simulink model "gnc_dst"  (R2023a)
settings: Solver=ode4  StartTime=0.0  StopTime=10.0  FixedStep=dt  RelTol=1e-3
undefined symbols (not defined in the file or in its folder): dt, plant, roe_mat, u_mat_full, u_time
libraries: aerolibutil x2
settings Model: Creator=ndelurgio  LastModifiedBy=ndelurgio
settings DebuggingCC: ModelReferenceExtraNoncontSigs=none

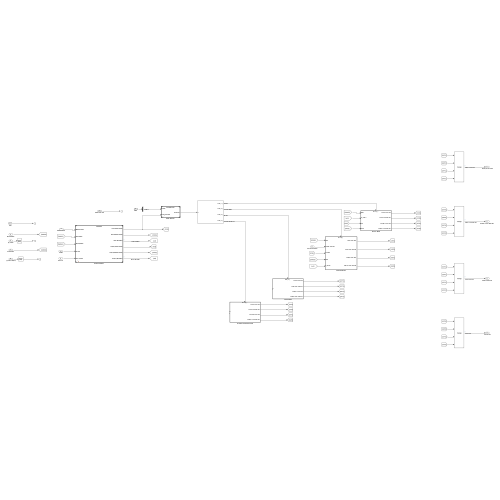
[thumbnail: Simulink's stored preview of the top-level diagram]
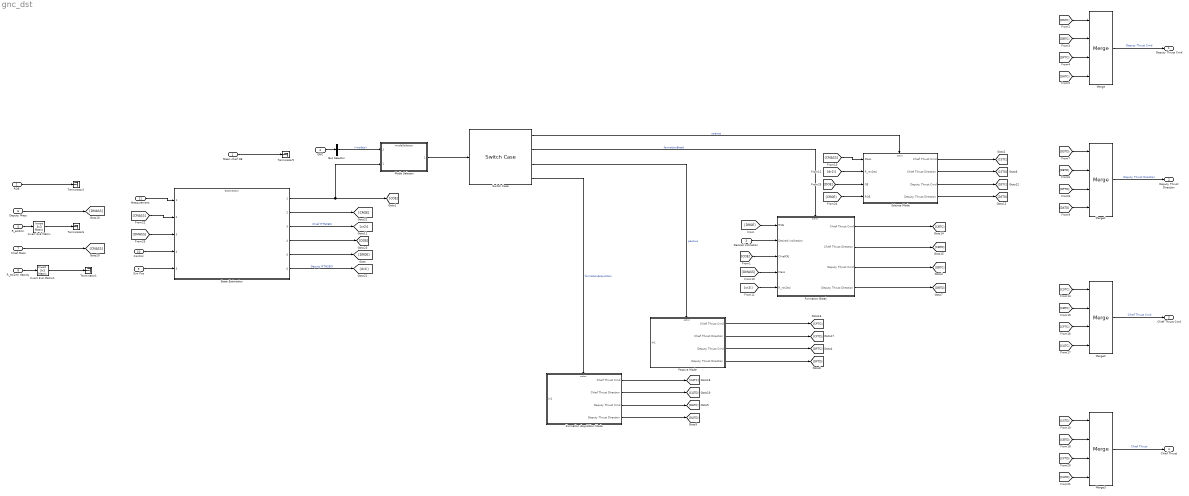
== system gnc_dst ==
  Mean chief OE : Inport  OutDataTypeStr=Bus: meanOrbitElements
  ROE : Inport  Port=2  OutDataTypeStr=Bus: eccentricSingularROE
  Desired inclination : Inport  Port=3  PortDimensions=2
  GNC : Inport  Port=4  OutDataTypeStr=Bus: gncBus
  R_eci2rtn : Inport  Port=5  PortDimensions=[3,3]
  Deputy Mass : Inport  Port=6
  Chief Mass : Inport  Port=7
  R_eci2rtn deputy : Inport  Port=8
  Sun Pos : Inport  Port=9
  Control : Inport  Port=10
  Measurement : Inport  Port=11
  Bus Selector : BusSelector  OutputSignals=modes
  Formation Acquisition Mode : Subsystem  TreatAsAtomicUnit=on
  Formation Break : Subsystem  TreatAsAtomicUnit=on
  Invert 3x3 Matrix : aerolibutil/Invert  3x3 Matrix
  Invert 3x3 Matrix1 : aerolibutil/Invert  3x3 Matrix
  Merge : Merge  Inputs=4  InitialOutput=0
  Merge1 : Merge  Inputs=4  InitialOutput=[1,1,1]
  Merge2 : Merge  Inputs=4  InitialOutput=0
  Merge3 : Merge  Inputs=4  InitialOutput=[1,1,1]
  Mode Selector : ModelReference  ModelNameDialog=modeSelector.slx  SimulationMode=Normal  ModelReferenceVersion=1.18
      settings: PortSchema="{\"entries\":[{\"content\":{\"sides\":[{\"content\":{\"connectorIds\":[\"In2\",\"In1\"]},\"type\":\"ConnectorPlacement.EquallySpacedRectSide\",\"uuid\":\"8a45dd05-9625-4267-a143-38565687985f\"},{\"content\":{\"connectorIds\":[\"Out1\"],\"side\":\"RIGHT\"},\"type\":\"ConnectorPlacement.EquallySpacedRectSide\",\"uuid\":\"c16609dd-c717-4d96-a97d-40d34aa61c5b\"},{\"content\":{\"side\":\"TOP\"},\"type\":\"ConnectorPlacement.EquallySpacedRectSide\",\"uuid\":\"265a618d-b5cc-4228-aeff-cbf882e13e2d\"}]},\"type\":\"ConnectorPlacement.EquallySpacedConnector\",\"uuid\":\"354b4fb0-049b-4d87-9ce4-a2a1b71aacc7\"}],\"packageUris\":[\"http://schema.mathworks.com/mf0/Connector/R2020b\"],\"version\":\"1.0\"}"
  Passive Mode : Subsystem  TreatAsAtomicUnit=on
  Science Mode : Subsystem  TreatAsAtomicUnit=on
  State Estimation : ModelReference  ModelNameDialog=estimation.slx  SimulationMode=Normal  ModelReferenceVersion=1.37
  Switch Case : SwitchCase  CaseConditions={1,2,3,4}  ShowDefaultCase=off
  Terminator{1..2,5..6} (4 alike) : Terminator
  Deputy Thrust Cmd : Outport
  Deputy Thrust Direction : Outport  Port=2
  Chief Thrust Cmd : Outport  Port=3
  Chief Thrust : Outport  Port=4
  wires:
  Mean chief OE/1 -> Terminator5/1
  ROE/1 -> Terminator2/1
  Desired inclination/1 -> Formation Break/2(Desired inclination)
  Merge/1 -> Deputy Thrust Cmd/1  "Deputy Thrust Cmd"
  Merge1/1 -> Deputy Thrust Direction/1  "Deputy Thrust Direction"
  Switch Case/1 -> Science Mode/Action  "science"
  Switch Case/2 -> Formation Break/Action  "formationBreak"
  Switch Case/3 -> Passive Mode/Action  "passive"
  Switch Case/4 -> Formation Acquisition Mode/Action  "formationAcquisition"
  Mode Selector/1 -> Switch Case/1
  GNC/1 -> Bus Selector/1
  Bus Selector/1 -> Mode Selector/2  "<modes>"
  [DROE] -> Formation Break/1(ROE)
  [COE] -> Formation Break/3(ChiefOE)
  Invert 3x3 Matrix/1 -> Terminator6/1
  Deputy Mass/1 -> [DMASS]
  R_eci2rtn/1 -> Invert 3x3 Matrix/1
  Science Mode/1(Chief Thrust Cmd) -> [CSTC]
  Formation Break/3(Deputy Thrust Cmd) -> [DBTC]
  Passive Mode/3(Deputy Thrust Cmd) -> [DPTC]
  Formation Acquisition Mode/3(Deputy Thrust Cmd) -> [DATC]
  [DSTC] -> Merge/1
  [DBTC] -> Merge/2
  [DPTC] -> Merge/3
  [DATC] -> Merge/4
  Science Mode/2(Chief Thrust Direction) -> [CSTD]
  Formation Break/4(Deputy Thrust Direction) -> [DBTD]
  Passive Mode/4(Deputy Thrust Direction) -> [DPTD]
  Formation Acquisition Mode/4(Deputy Thrust Direction) -> [DATD]
  [DSTD] -> Merge1/1
  [DBTD] -> Merge1/2
  [DPTD] -> Merge1/3
  [DATD] -> Merge1/4
  [DMASS] -> Formation Break/4(Mass)
  [cr2i] -> Formation Break/5(R_rtn2eci)
  [dr2i] -> Science Mode/2(R_rtn2eci)
  [CMASS] -> Science Mode/1(Mass)
  Science Mode/3(Deputy Thrust Cmd) -> [DSTC]
  Science Mode/4(Deputy Thrust Direction) -> [DSTD]
  Formation Break/2(Chief Thrust Direction) -> [CBTD]
  Formation Break/1(Chief Thrust Cmd) -> [CBTC]
  Passive Mode/1(Chief Thrust Cmd) -> [CPTC]
  Passive Mode/2(Chief Thrust Direction) -> [CPTD]
  Formation Acquisition Mode/1(Chief Thrust Cmd) -> [CATC]
  Formation Acquisition Mode/2(Chief Thrust Direction) -> [CATD]
  [CSTC] -> Merge2/1
  [CPTC] -> Merge2/3
  [CATC] -> Merge2/4
  [CBTC] -> Merge2/2
  [CSTD] -> Merge3/1
  [CBTD] -> Merge3/2
  [CATD] -> Merge3/4
  [CPTD] -> Merge3/3
  Merge3/1 -> Chief Thrust/1  "Chief Thrust"
  Merge2/1 -> Chief Thrust Cmd/1  "Chief Thrust Cmd"
  Chief Mass/1 -> [CMASS]
  R_eci2rtn deputy/1 -> Invert 3x3 Matrix1/1
  Invert 3x3 Matrix1/1 -> Terminator1/1
  [CMASS] -> State Estimation/2
  [DMASS] -> State Estimation/3
  Sun Pos/1 -> State Estimation/5
  Control/1 -> State Estimation/4
  Measurement/1 -> State Estimation/1
  State Estimation/1 -> Mode Selector/1, [COE]
  State Estimation/2 -> [CROE]
  State Estimation/3 -> [cr2i]  "Chief RTN2ECI"
  State Estimation/4 -> [DOE]
  State Estimation/5 -> [DROE]
  State Estimation/6 -> [dr2i]  "Deputy RTN2ECI"
  [CROE] -> Science Mode/4(ROE)
  [DOE] -> Science Mode/3(OE)

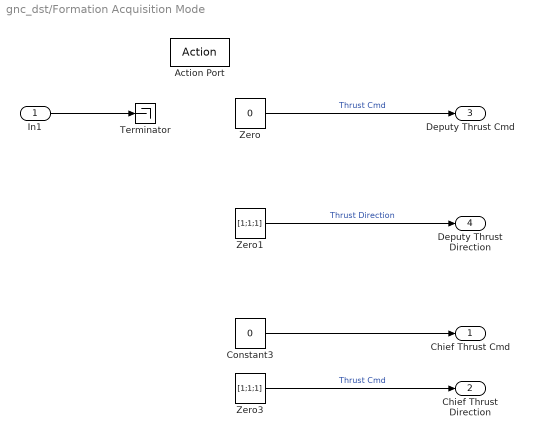
== system gnc_dst/Formation Acquisition Mode ==
  In1 : Inport
  Action Port : ActionPort  ActionPortLabel=case [ 4 ]:
  Constant3 : Constant  Value=0
  Terminator : Terminator
  Zero : Constant  Value=0  OutDataTypeStr=Inherit: Inherit via back propagation
  Zero1 : Constant  Value=[1;1;1]  OutDataTypeStr=Inherit: Inherit via back propagation
  Zero3 : Constant  Value=[1;1;1]  OutDataTypeStr=Inherit: Inherit via back propagation
  Chief Thrust Cmd : Outport
  Chief Thrust Direction : Outport  Port=2
  Deputy Thrust Cmd : Outport  Port=3
  Deputy Thrust Direction : Outport  Port=4
  wires:
  In1/1 -> Terminator/1
  Zero/1 -> Deputy Thrust Cmd/1  "Thrust Cmd"
  Zero1/1 -> Deputy Thrust Direction/1  "Thrust Direction"
  Zero3/1 -> Chief Thrust Direction/1  "Thrust Cmd"
  Constant3/1 -> Chief Thrust Cmd/1

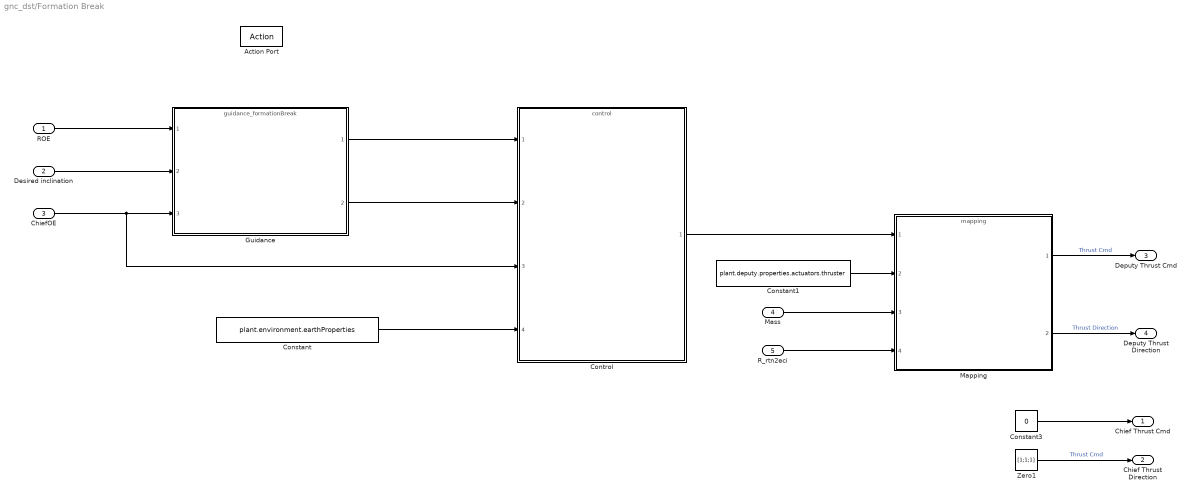
== system gnc_dst/Formation Break ==
  ROE : Inport
  Desired inclination : Inport  Port=2
  ChiefOE : Inport  Port=3
  Mass : Inport  Port=4
  R_rtn2eci : Inport  Port=5
  Action Port : ActionPort  ActionPortLabel=case [ 2 ]:
  Constant : Constant  Value=plant.environment.earthProperties  OutDataTypeStr=Bus: earthProperties
  Constant1 : Constant  Value=plant.deputy.properties.actuators.thruster  OutDataTypeStr=Bus: thruster
  Constant3 : Constant  Value=0
  Control : ModelReference  ModelNameDialog=control.slx  SimulationMode=Normal  ModelReferenceVersion=1.14
  Guidance : ModelReference  ModelNameDialog=guidance_formationBreak  SimulationMode=Normal  ModelReferenceVersion=1.56
  Mapping : ModelReference  ModelNameDialog=mapping.slx  SimulationMode=Normal  ModelReferenceVersion=1.29
  Zero1 : Constant  Value=[1;1;1]  OutDataTypeStr=Inherit: Inherit via back propagation
  Chief Thrust Cmd : Outport
  Chief Thrust Direction : Outport  Port=2
  Deputy Thrust Cmd : Outport  Port=3
  Deputy Thrust Direction : Outport  Port=4
  wires:
  ROE/1 -> Guidance/1
  Guidance/1 -> Control/1
  Guidance/2 -> Control/2
  Desired inclination/1 -> Guidance/2
  ChiefOE/1 -> Control/3, Guidance/3
  Constant/1 -> Control/4
  Control/1 -> Mapping/1
  Constant1/1 -> Mapping/2
  Mass/1 -> Mapping/3
  R_rtn2eci/1 -> Mapping/4
  Mapping/1 -> Deputy Thrust Cmd/1  "Thrust Cmd"
  Mapping/2 -> Deputy Thrust Direction/1  "Thrust Direction"
  Constant3/1 -> Chief Thrust Cmd/1
  Zero1/1 -> Chief Thrust Direction/1  "Thrust Cmd"

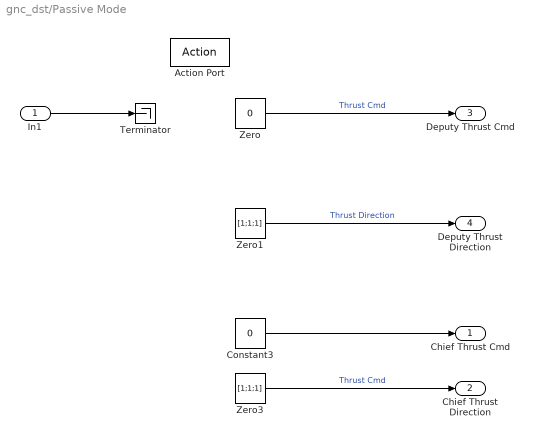
== system gnc_dst/Passive Mode ==
  In1 : Inport
  Action Port : ActionPort  ActionPortLabel=case [ 3 ]:
  Constant3 : Constant  Value=0
  Terminator : Terminator
  Zero : Constant  Value=0  OutDataTypeStr=Inherit: Inherit via back propagation
  Zero1 : Constant  Value=[1;1;1]  OutDataTypeStr=Inherit: Inherit via back propagation
  Zero3 : Constant  Value=[1;1;1]  OutDataTypeStr=Inherit: Inherit via back propagation
  Chief Thrust Cmd : Outport
  Chief Thrust Direction : Outport  Port=2
  Deputy Thrust Cmd : Outport  Port=3
  Deputy Thrust Direction : Outport  Port=4
  wires:
  In1/1 -> Terminator/1
  Zero/1 -> Deputy Thrust Cmd/1  "Thrust Cmd"
  Zero1/1 -> Deputy Thrust Direction/1  "Thrust Direction"
  Zero3/1 -> Chief Thrust Direction/1  "Thrust Cmd"
  Constant3/1 -> Chief Thrust Cmd/1

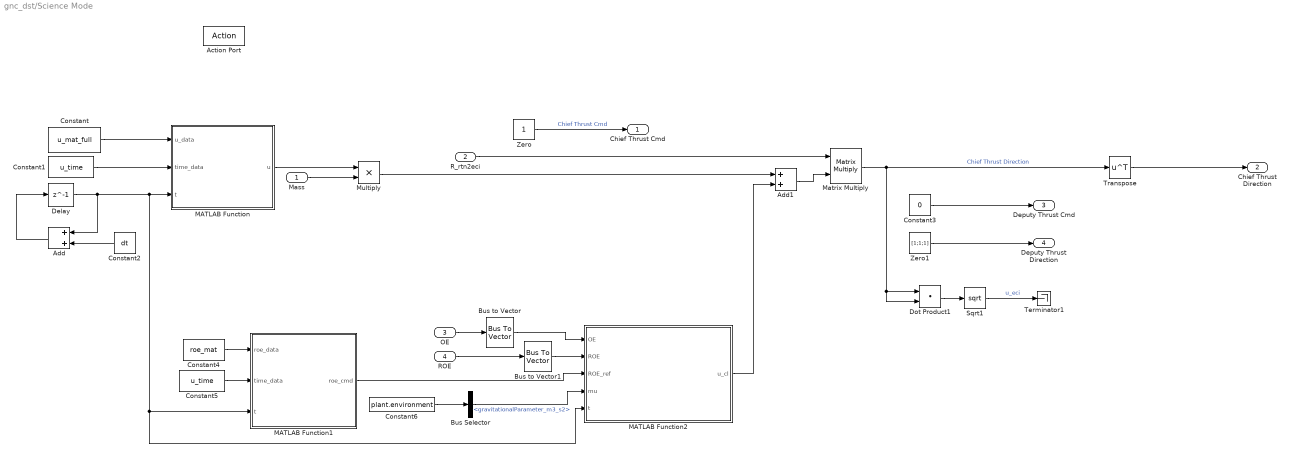
== system gnc_dst/Science Mode ==
  Mass : Inport
  R_rtn2eci : Inport  Port=2
  OE : Inport  Port=3  OutDataTypeStr=Bus: osculatingOrbitElements
  ROE : Inport  Port=4  OutDataTypeStr=Bus: eccentricSingularROE
  Action Port : ActionPort  ActionPortLabel=case [ 1 ]:
  Add : Sum
  Add1 : Sum
  Bus Selector : BusSelector  OutputSignals=earthProperties.gravitationalParameter_m3_s2
  Bus to Vector : BusToVector
  Bus to Vector1 : BusToVector
  Constant : Constant  Value=u_mat_full
  Constant1 : Constant  Value=u_time
  Constant2 : Constant  Value=dt
  Constant3 : Constant  Value=0
  Constant4 : Constant  Value=roe_mat
  Constant5 : Constant  Value=u_time
  Constant6 : Constant  Value=plant.environment  OutDataTypeStr=Bus: environment
  Delay : Delay  DelayLength=1
  Dot Product1 : DotProduct  OutDataTypeStr=Inherit: Inherit via internal rule
  MATLAB Function : MATLAB Function  TreatAsAtomicUnit=on
  MATLAB Function1 : MATLAB Function  TreatAsAtomicUnit=on
  MATLAB Function2 : MATLAB Function  TreatAsAtomicUnit=on
  Matrix Multiply : Product  Multiplication=Matrix(*)
  Multiply : Product  Inputs=**
  Sqrt1 : Sqrt
  Terminator1 : Terminator
  Transpose : Math  Operator=transpose
  Zero : Constant  OutDataTypeStr=Inherit: Inherit via back propagation
  Zero1 : Constant  Value=[1;1;1]  OutDataTypeStr=Inherit: Inherit via back propagation
  Chief Thrust Cmd : Outport
  Chief Thrust Direction : Outport  Port=2
  Deputy Thrust Cmd : Outport  Port=3
  Deputy Thrust Direction : Outport  Port=4
  wires:
  Zero/1 -> Chief Thrust Cmd/1  "Chief Thrust Cmd"
  Constant/1 -> MATLAB Function/1(u_data)
  Constant1/1 -> MATLAB Function/2(time_data)
  Delay/1 -> Add/1, MATLAB Function1/3(t), MATLAB Function2/5(t), MATLAB Function/3(t)
  Constant2/1 -> Add/2
  Add/1 -> Delay/1
  MATLAB Function/1(u) -> Multiply/1
  Mass/1 -> Multiply/2
  R_rtn2eci/1 -> Matrix Multiply/1
  Multiply/1 -> Add1/1
  Constant3/1 -> Deputy Thrust Cmd/1
  Zero1/1 -> Deputy Thrust Direction/1
  Matrix Multiply/1 -> Dot Product1/2, Dot Product1/1, Transpose/1  "Chief Thrust Direction"
  Dot Product1/1 -> Sqrt1/1
  Sqrt1/1 -> Terminator1/1  "u_eci"
  Transpose/1 -> Chief Thrust Direction/1
  Constant4/1 -> MATLAB Function1/1(roe_data)
  Constant5/1 -> MATLAB Function1/2(time_data)
  MATLAB Function1/1(roe_cmd) -> MATLAB Function2/3(ROE_ref)
  OE/1 -> Bus to Vector/1
  ROE/1 -> Bus to Vector1/1
  Constant6/1 -> Bus Selector/1
  Bus Selector/1 -> MATLAB Function2/4(mu)  "<gravitationalParameter_m3_s2>"
  MATLAB Function2/1(u_cl) -> Add1/2
  Add1/1 -> Matrix Multiply/2
  Bus to Vector/1 -> MATLAB Function2/1(OE)
  Bus to Vector1/1 -> MATLAB Function2/2(ROE)

== matlab function gnc_dst/Science Mode/MATLAB Function1 ==
  data: roe_data input; roe_cmd output; time_data input; t input
function roe_cmd = getROECmd(roe_data,time_data,t)

roe_cmd = getROECmd(roe_data,time_data,t);

end

== matlab function gnc_dst/Science Mode/MATLAB Function ==
  data: u_data input; u output; time_data input; t input
function u = getControlCmd(u_data,time_data,t)
u = getControlCmd(u_data,time_data,t);
end

== matlab function gnc_dst/Science Mode/MATLAB Function2 ==
  data: OE input; u_cl output; ROE input; ROE_ref input; mu input; t input
function u_cl = getClosedLoopCmd(OE,ROE,ROE_ref,mu,t)

if t > 900 && t < 19080
    u_cl = getClosedLoopCmd(OE,ROE,ROE_ref,mu);
else
    u_cl = [0;0;0];

end
